simulink model "CSD_Segway_hardware"  (R2018b)
settings: Solver=ode5  StartTime=0.0  StopTime=10.0  FixedStep=1e-4  RelTol=1e-3
values from neighbouring files (symbols this model uses):
  K = place(A, B, 1e2*[-5,      -1, -0.8, -0.8,      -2e-2, -2e-2])    [CSD_project.m]
  R = 0.028    [CSD_project.m]
  W = 0.126    [CSD_project.m]
undefined symbols (not defined in the file or in its folder): DiscIntNeverNeededParam
libraries: legoev3lib x5, simulink x1, dspfdesign x1
settings Model: Creator=sh  LastModifiedBy=shiha

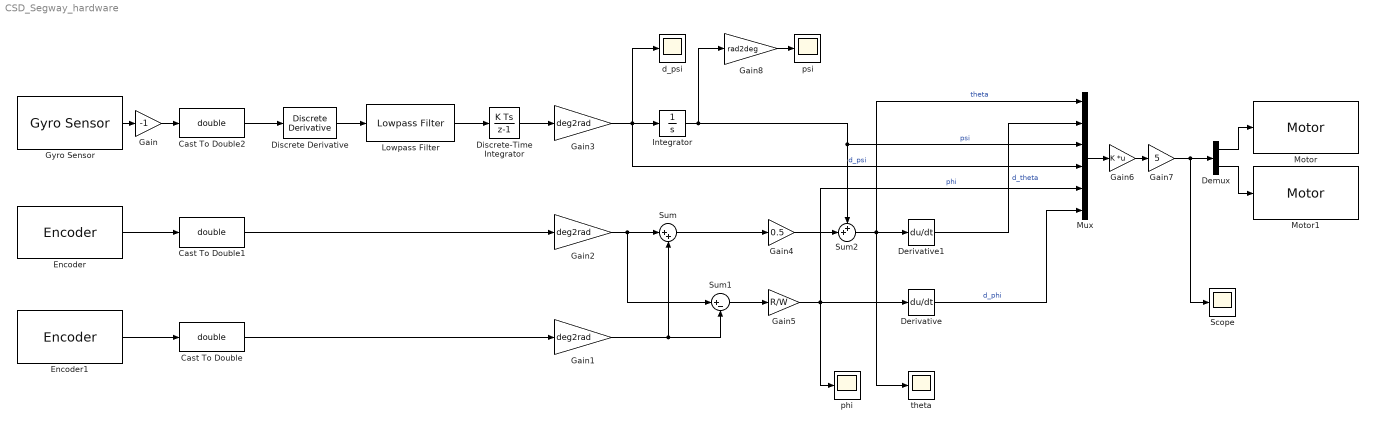
== system CSD_Segway_hardware ==
  Cast To Double : DataTypeConversion  OutDataTypeStr=double
  Cast To Double1 : DataTypeConversion  OutDataTypeStr=double
  Cast To Double2 : DataTypeConversion  OutDataTypeStr=double
  Demux : Demux  Outputs=2
  Derivative : Derivative
  Derivative1 : Derivative
  Discrete Derivative : simulink/Discrete/Discrete Derivative  gainval=1.0  ICPrevScaledInput=0.0  OutMin=[]  OutMax=[]  OutDataType=fixdt(1, 16)  OutScaling=2^-10  DoSatur=off
  Discrete-Time Integrator : DiscreteIntegrator  SampleTime=-1  ICPrevOutput=DiscIntNeverNeededParam  ICPrevScaledInput=DiscIntNeverNeededParam
  Encoder : legoev3lib/Encoder  portNumber=A  opMode=No reset  sampleTime=4e-3
      settings: SourceProductName=Simulink Support Package for LEGO MINDSTORMS EV3 Hardware  SourceProductBaseCode=LEGOEV3
  Encoder1 : legoev3lib/Encoder  portNumber=B  opMode=No reset  sampleTime=4e-3
      settings: SourceProductName=Simulink Support Package for LEGO MINDSTORMS EV3 Hardware  SourceProductBaseCode=LEGOEV3
  Gain : Gain  Gain=-1
  Gain1 : Gain  Gain=deg2rad
  Gain2 : Gain  Gain=deg2rad
  Gain3 : Gain  Gain=deg2rad
  Gain4 : Gain  Gain=0.5
  Gain5 : Gain  Gain=R/W
  Gain6 : Gain  Gain=K  Multiplication=Matrix(K*u)
  Gain7 : Gain  Gain=5
  Gain8 : Gain  Gain=rad2deg
  Gyro Sensor : legoev3lib/Gyro Sensor  portNumber=1  sampleTime=4e-3
      settings: SourceProductName=Simulink Support Package for LEGO MINDSTORMS EV3 Hardware  SourceProductBaseCode=LEGOEV3
  Integrator : Integrator  InitialCondition=pi/36
  Lowpass Filter : dspfdesign/Lowpass Filter  FilterType=FIR  DesignForMinimumOrder=on  FilterOrder=50  PassbandFrequency=8e3  StopbandFrequency=12e3  PassbandRipple=0.1  StopbandAttenuation=80  InheritSampleRate=off  SampleRate=44100  SimulateUsing=Interpreted execution  roundingMode=Floor  coeffsDataTypeStr=fixdt(1,16)
  Motor : legoev3lib/Motor  sportNumber=A  sstopAction=Brake
  Motor1 : legoev3lib/Motor  sportNumber=B  sstopAction=Brake
  Mux : Mux  Inputs=6
  Scope : Scope
  Sum : Sum  Inputs=|++
  Sum1 : Sum  Inputs=|+-
  Sum2 : Sum  Inputs=++|
  d_psi : Scope
  phi : Scope
  psi : Scope
  theta : Scope
  wires:
  Encoder1/1 -> Cast To Double/1
  Encoder/1 -> Cast To Double1/1
  Gyro Sensor/1 -> Gain/1
  Gain/1 -> Cast To Double2/1
  Cast To Double2/1 -> Discrete Derivative/1
  Cast To Double1/1 -> Gain2/1
  Cast To Double/1 -> Gain1/1
  Gain3/1 -> Mux/4, d_psi/1, Integrator/1  "d_psi"
  Discrete Derivative/1 -> Lowpass Filter/1
  Lowpass Filter/1 -> Discrete-Time Integrator/1
  Discrete-Time Integrator/1 -> Gain3/1
  Integrator/1 -> Mux/3, Sum2/1, Gain8/1  "psi"
  Gain2/1 -> Sum1/1, Sum/1
  Gain1/1 -> Sum1/2, Sum/2
  Sum/1 -> Gain4/1
  Sum1/1 -> Gain5/1
  Gain5/1 -> Mux/5, phi/1, Derivative/1  "phi"
  Gain4/1 -> Sum2/2
  Sum2/1 -> Mux/1, theta/1, Derivative1/1  "theta"
  Derivative1/1 -> Mux/2  "d_theta"
  Derivative/1 -> Mux/6  "d_phi"
  Mux/1 -> Gain6/1
  Gain6/1 -> Gain7/1
  Demux/1 -> Motor/1
  Demux/2 -> Motor1/1
  Gain7/1 -> Scope/1, Demux/1
  Gain8/1 -> psi/1
